simulink model "sim_1d_kalman"  (R2023b)
settings: Solver=VariableStepAuto  StartTime=0.0  StopTime=10.0  RelTol=1e-3
settings Model: Creator=Jhchen  LastModifiedBy=Jhchen

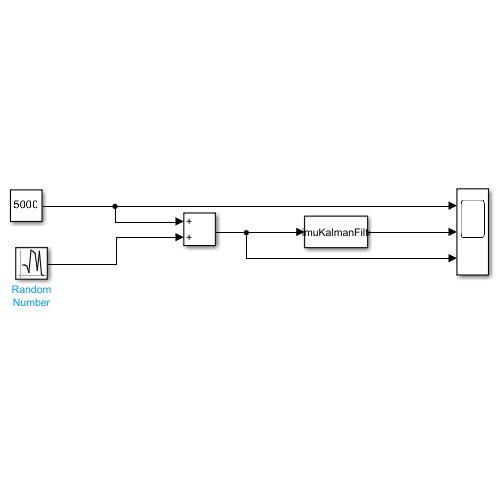
[thumbnail: Simulink's stored preview of the top-level diagram]
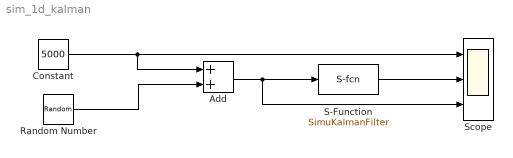
== system sim_1d_kalman ==
  Add : Sum
  Constant : Constant  Value=5000
  Random Number : RandomNumber  Variance=5  SampleTime=0.1
  S-Function : S-Function  FunctionName=SimuKalmanFilter  SFunctionDeploymentMode=off  EnableBusSupport=off
  Scope : Scope  NumInputPorts=3
  wires:
  S-Function/1 -> Scope/2
  Add/1 -> Scope/3, S-Function/1
  Constant/1 -> Add/1, Scope/1
  Random Number/1 -> Add/2
